simulink model "UPFC"  (R2021a)
settings: Solver=ode45  StartTime=0.0  StopTime=1  RelTol=1e-3  EnableMultiTasking=on
undefined symbols (not defined in the file): D1, Delta
libraries: spsThreePhaseVIMeasurementLib x9, spsMosfetLib x6, spsThyristorLib x6, spsVoltageMeasurementLib x3, spsThreePhaseBreakerLib x2, spsThreePhaseTransformerInductanceMatrixTypeTwoWindingsLib x2, spsCurrentMeasurementLib x1, spsSeriesRLCBranchLib x1, spsDistributedParametersLineLib x1, spsThreePhaseSourceLib x1, spspowerguiLib x1
settings Model: Creator=Indhu  LastModifiedBy=Rahul
settings SolverCC: AlgebraicLoopSolver=TrustRegion
settings DataIOCC: LimitDataPoints=on  SaveFormat=Array  ReturnWorkspaceOutputs=off
settings OptimizationCC: LifeSpan=inf
settings DebuggingCC: SolverPrmCheckMsg=warning  SFUnexpectedBacktrackingDiag=warning  SFNoUnconditionalDefaultTransitionDiag=warning  SFExecutionAtInitializationDiag=none  SFMachineParentedDataDiag=warning  ArithmeticOperatorsInVariantConditions=warning
settings HardwareCC: ProdBitPerPointer=32  ProdBitPerSizeT=32  ProdBitPerPtrDiffT=32  ProdLargestAtomicFloat=None  ProdIntDivRoundTo=Undefined  ProdEndianess=Unspecified  ProdWordSize=32  ProdHWDeviceType=32-bit Generic
settings ModelReferenceCC: PropagateSignalLabelsOutOfModel=off
settings SFSimCC: SimUseLocalCustomCode=off  CustomCodeUndefinedFunction=UseInterfaceOnly
settings RTWCC: RTWUseLocalCustomCode=off
settings CodeAppCC: StateflowObjectComments=on
settings GRTTargetCC: TargetLangStandard=C89/C90 (ANSI)
settings ConfigComp: CovMetricSettings=dw  CovSaveCumulativeToWorkspaceVar=on  CovSaveSingleToWorkspaceVar=on  CovExternalEMLEnable=off  CovSFcnEnable=off
settings SimscapeCC: SimscapeNormalizeSystem=off

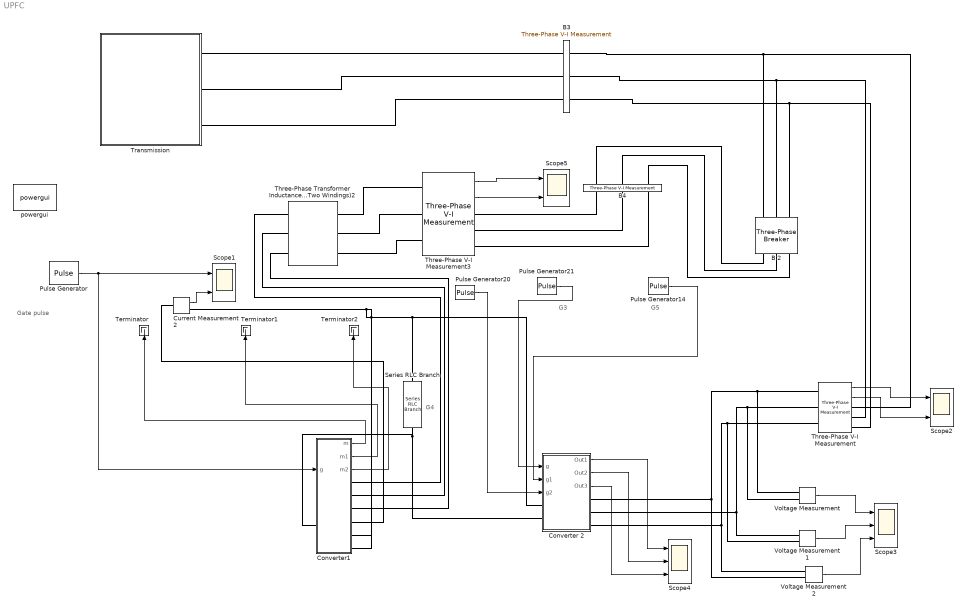
== system UPFC ==
  note: G4
  note: G5
  note: G3
  note: Gate pulse
  B 2 : spsThreePhaseBreakerLib/Three-Phase Breaker  InitialState=closed  SwitchA=off  SwitchB=off  SwitchC=off  SwitchTimes="[1/50  20/50]"  External=off  BreakerResistance=0.001  SnubberResistance=1e6  SnubberCapacitance=inf  Measurements=None
  B3 : spsThreePhaseVIMeasurementLib/Three-Phase V-I Measurement  VoltageMeasurement=phase-to-ground  SetLabelV=on  LabelV=Vabc_B3  Vpu=off  VpuLL=off  CurrentMeasurement=no  SetLabelI=off  LabelI=A1  Ipu=off  Pbase=100e6  Vbase=440  OutputType=Magnitude  PhasorSimulation=off  PSBequivalent=0
  B4 : spsThreePhaseVIMeasurementLib/Three-Phase V-I Measurement  VoltageMeasurement=phase-to-phase  SetLabelV=on  LabelV=Vabc_B4  Vpu=off  VpuLL=off  CurrentMeasurement=yes  SetLabelI=on  LabelI=Iabc_B4  Ipu=off  Pbase=100e6  Vbase=440  OutputType=Magnitude  PhasorSimulation=off  PSBequivalent=0
  Converter 2 : Subsystem
  Converter1 : Subsystem
  Current Measurement2 : spsCurrentMeasurementLib/Current Measurement  PhasorSimulation=off  OutputType=Complex  PSBequivalent=0
  Pulse Generator : DiscretePulseGenerator  PulseType=Time based  Amplitude=10  Period=0.02/3  PulseWidth=20  PhaseDelay=0.0025
  Pulse Generator14 : DiscretePulseGenerator  PulseType=Time based  Period=0.02  PulseWidth=50  PhaseDelay=0.04/3
  Pulse Generator20 : DiscretePulseGenerator  PulseType=Time based  Period=0.02  PulseWidth=50
  Pulse Generator21 : DiscretePulseGenerator  PulseType=Time based  Period=0.02  PulseWidth=50  PhaseDelay=0.02/3
  Scope1 : Scope  NumInputPorts=2
  Scope2 : Scope  NumInputPorts=2
  Scope3 : Scope  NumInputPorts=3
  Scope4 : Scope  NumInputPorts=3
  Scope5 : Scope  NumInputPorts=2
  Series RLC Branch : spsSeriesRLCBranchLib/Series RLC Branch  LConnTagsString=__new0  RConnTagsString=__new0  BranchType=C  Resistance=1  Inductance=1e-3  SetiL0=off  InitialCurrent=0  Capacitance=10  Setx0=off  InitialVoltage=0  Measurements=None
  Terminator : Terminator
  Terminator1 : Terminator
  Terminator2 : Terminator
  Three-Phase V-I Measurement : spsThreePhaseVIMeasurementLib/Three-Phase V-I Measurement  VoltageMeasurement=phase-to-ground  SetLabelV=off  LabelV=Vabc  Vpu=off  VpuLL=off  CurrentMeasurement=yes  SetLabelI=off  LabelI=Iabc  Ipu=off  Pbase=100e6  Vbase=500e3  OutputType=Complex  PhasorSimulation=off  PSBequivalent=0
  Three-Phase V-I Measurement3 : spsThreePhaseVIMeasurementLib/Three-Phase V-I Measurement  VoltageMeasurement=phase-to-phase  SetLabelV=off  LabelV=Vabc  Vpu=off  VpuLL=off  CurrentMeasurement=yes  SetLabelI=off  LabelI=Iabc  Ipu=off  Pbase=100e6  Vbase=500e3  OutputType=Complex  PhasorSimulation=off  PSBequivalent=0
  Three-Phase Transformer Inductance Matrix Type (Two Windings)2 : spsThreePhaseTransformerInductanceMatrixTypeTwoWindingsLib/Three-Phase Transformer Inductance Matrix Type (Two Windings)  CoreType=Three-limb or five-limb core  Winding1Connection=Delta (D1)  Winding2Connection=Yg  AutoTransformer=off  Measurements=None  NominalPower=[100e3 50]  VLLnom=[254.03 254.03]  WindingResistances=[0.01 0.01]  NoLoadIexcPos=2  NoLoadPlossPos=1000  ShortCircuitReactancePos=0.06  ShortCircuitReactancePosAuto=0.06  NoLoadIexcZero=100  NoLoadPlossZero=1500  ShortCircuitReactanceZero=0.03  ShortCircuitReactanceZeroAuto=0.03
      settings: SourceProductBaseCode=PS
  "Transmission " : Subsystem
  Voltage Measurement : spsVoltageMeasurementLib/Voltage Measurement  PhasorSimulation=off  OutputType=Complex  PSBequivalent=0
  Voltage Measurement1 : spsVoltageMeasurementLib/Voltage Measurement  PhasorSimulation=off  OutputType=Complex  PSBequivalent=0
  Voltage Measurement2 : spsVoltageMeasurementLib/Voltage Measurement  PhasorSimulation=off  OutputType=Complex  PSBequivalent=0
  powergui : spspowerguiLib/powergui  Priority=1  SimulationMode=Discrete  SampleTime=50e-6  frequency=60  Iterations=50  frequencyindice=50  Pbase=100e6  ErrMax=1e-4  UnitsV=kV  UnitsW=MW  buscounter=0  FunctionMessages=off  echomessages=off  EnableUseOfTLC=off  CurrentSourceSwitches=off  DisableSnubberDevices=off  DisableRonSwitches=off  DisableVfSwitches=off  DisplayEquations=off  AutomaticDiscreteSolvers=off  SolverType=Tustin  Interpol=off  ExternalGateDelay=off  methode=off  Ts=0  x0status=blocks  SPID=off  SwTol=0  HookPort=off  NonlinearTolerance=1e-4  nMaxIteration=100  ContinueOnMaxIteration=off  RestoreLinks=warning  ResistiveCurrentMeasurement=off  Frange=[0:2:500]  Ylog=off  Xlog=on  ShowGrid=off  save=off  variable=ZData  structure=0  ZoomFFT=off  StartTime=0.0  cycles=1  DisplayStyle=1  fundamental=60  FreqAxis=off  MaxFrequency=1000  frequencyindicesteady=1  RmsSteady=1  display=off
  wires:
  Pulse Generator/1 -> Converter1/1(g), Scope1/1
  Current Measurement2/1 -> Scope1/2
  Three-Phase V-I Measurement/2 -> Scope2/2
  Three-Phase V-I Measurement/1 -> Scope2/1
  Voltage Measurement/1 -> Scope3/1
  Voltage Measurement1/1 -> Scope3/2
  Voltage Measurement2/1 -> Scope3/3
  Three-Phase V-I Measurement3/1 -> Scope5/1
  Three-Phase V-I Measurement3/2 -> Scope5/2
  Converter1/1(m) -> Terminator/1
  Converter1/2(m1) -> Terminator1/1
  Converter1/3(m2) -> Terminator2/1
  Pulse Generator21/1 -> Converter 2/1(g)
  Pulse Generator14/1 -> Converter 2/2(g1)
  Pulse Generator20/1 -> Converter 2/3(g2)
  Converter 2/1(Out1) -> Scope4/1
  Converter 2/2(Out2) -> Scope4/2
  Converter 2/3(Out3) -> Scope4/3
  connections:
  Current Measurement2/RConn1 -- Converter1/RConn5 -- Converter1/RConn6 -- Converter 2/LConn1 -- Series RLC Branch/LConn1
  Series RLC Branch/RConn1 -- Converter 2/LConn2 -- Converter1/LConn1
  Voltage Measurement1/LConn1 -- Voltage Measurement/LConn2 -- Three-Phase V-I Measurement/LConn2 -- Converter 2/RConn2
  B3/LConn3 -- Three-Phase V-I Measurement/RConn3 -- B 2/LConn3
  B3/LConn1 -- Three-Phase V-I Measurement/RConn1 -- B 2/LConn1
  B3/LConn2 -- Three-Phase V-I Measurement/RConn2 -- B 2/LConn2
  Three-Phase V-I Measurement3/RConn3 -- B4/RConn3
  B4/LConn1 -- B 2/RConn1
  B4/LConn3 -- B 2/RConn3
  Three-Phase V-I Measurement3/RConn1 -- B4/RConn1
  Three-Phase V-I Measurement3/RConn2 -- B4/RConn2
  B4/LConn2 -- B 2/RConn2
  Three-Phase V-I Measurement3/LConn1 -- Three-Phase Transformer Inductance Matrix Type (Two Windings)2/RConn1
  Three-Phase V-I Measurement3/LConn2 -- Three-Phase Transformer Inductance Matrix Type (Two Windings)2/RConn2
  Three-Phase V-I Measurement3/LConn3 -- Three-Phase Transformer Inductance Matrix Type (Two Windings)2/RConn3
  Three-Phase Transformer Inductance Matrix Type (Two Windings)2/LConn1 -- Converter1/RConn1
  Three-Phase Transformer Inductance Matrix Type (Two Windings)2/LConn2 -- Converter1/RConn2
  Three-Phase Transformer Inductance Matrix Type (Two Windings)2/LConn3 -- Converter1/RConn3
  Current Measurement2/LConn1 -- Converter1/RConn4
  Voltage Measurement2/LConn2 -- Voltage Measurement/LConn1 -- Three-Phase V-I Measurement/LConn1 -- Converter 2/RConn1
  Voltage Measurement1/LConn2 -- Voltage Measurement2/LConn1 -- Converter 2/RConn3 -- Three-Phase V-I Measurement/LConn3
  "Transmission "/RConn1 -- B3/RConn1
  "Transmission "/RConn2 -- B3/RConn2
  "Transmission "/RConn3 -- B3/RConn3

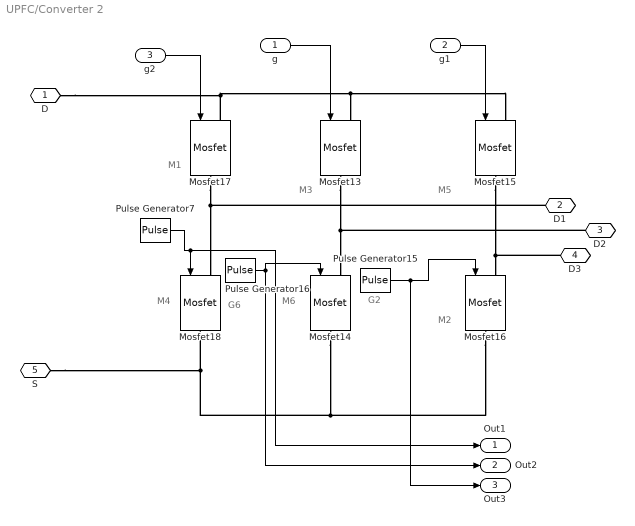
== system UPFC/Converter 2 ==
  note: M1
  note: M2
  note: M4
  note: M6
  note: M3
  note: M5
  note: G6
  note: G2
  g : Inport
  g1 : Inport  Port=2
  g2 : Inport  Port=3
  Mosfet{13..18} (6 alike) : spsMosfetLib/Mosfet  Ron=0.001  Lon=1e-6  Rd=.001  Vfd=0  IC=0  Rs=1e5  Cs=inf  Measurements=off
  Pulse Generator15 : DiscretePulseGenerator  PulseType=Time based  Period=0.02  PulseWidth=50  PhaseDelay=0.01/3
  Pulse Generator16 : DiscretePulseGenerator  PulseType=Time based  Period=0.02  PulseWidth=50  PhaseDelay=0.05/3
  Pulse Generator7 : DiscretePulseGenerator  PulseType=Time based  Period=0.02  PulseWidth=50  PhaseDelay=0.01
  D : PMIOPort  Side=Left
  D1 : PMIOPort  Port=2  Side=Right
  D2 : PMIOPort  Port=3  Side=Right
  D3 : PMIOPort  Port=4  Side=Right
  S : PMIOPort  Port=5  Side=Left
  Out1 : Outport
  Out2 : Outport  Port=2
  Out3 : Outport  Port=3
  wires:
  Pulse Generator7/1 -> Out1/1, Mosfet18/1
  Pulse Generator15/1 -> Out3/1, Mosfet16/1
  g1/1 -> Mosfet15/1
  Pulse Generator16/1 -> Out2/1, Mosfet14/1
  g/1 -> Mosfet13/1
  g2/1 -> Mosfet17/1
  connections:
  Mosfet17/LConn1 -- Mosfet15/LConn1 -- Mosfet13/LConn1 -- D/RConn1
  Mosfet16/RConn1 -- S/RConn1 -- Mosfet18/RConn1 -- Mosfet14/RConn1
  Mosfet17/RConn1 -- D1/RConn1 -- Mosfet18/LConn1
  Mosfet13/RConn1 -- D2/RConn1 -- Mosfet14/LConn1
  Mosfet15/RConn1 -- D3/RConn1 -- Mosfet16/LConn1

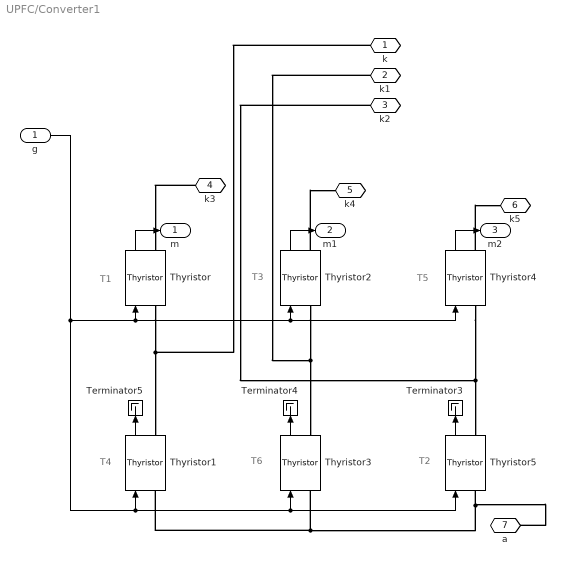
== system UPFC/Converter1 ==
  note: T1
  note: T4
  note: T3
  note: T5
  note: T6
  note: T2
  g : Inport
  Terminator3 : Terminator
  Terminator4 : Terminator
  Terminator5 : Terminator
  Thyristor{,1..5} (6 alike) : spsThyristorLib/Thyristor  Ron=0.001  Lon=0  Vf=0.8  IC=0  Rs=500  Cs=250e-9  Measurements=on
  k : PMIOPort  Side=Right
  k1 : PMIOPort  Port=2  Side=Right
  k2 : PMIOPort  Port=3  Side=Right
  k3 : PMIOPort  Port=4  Side=Right
  k4 : PMIOPort  Port=5  Side=Right
  k5 : PMIOPort  Port=6  Side=Right
  a : PMIOPort  Port=7  Side=Left
  m : Outport
  m1 : Outport  Port=2
  m2 : Outport  Port=3
  wires:
  Thyristor3/1 -> Terminator4/1
  Thyristor5/1 -> Terminator3/1
  g/1 -> Thyristor1/1, Thyristor5/1, Thyristor3/1, Thyristor/1, Thyristor2/1, Thyristor4/1
  Thyristor1/1 -> Terminator5/1
  Thyristor4/1 -> m2/1
  Thyristor/1 -> m/1
  Thyristor2/1 -> m1/1
  connections:
  Thyristor4/LConn1 -- k2/RConn1 -- Thyristor5/RConn1
  Thyristor5/LConn1 -- Thyristor1/LConn1 -- Thyristor3/LConn1 -- a/RConn1
  Thyristor2/LConn1 -- k1/RConn1 -- Thyristor3/RConn1
  Thyristor/LConn1 -- k/RConn1 -- Thyristor1/RConn1
  k3/RConn1 -- Thyristor/RConn1
  Thyristor2/RConn1 -- k4/RConn1
  Thyristor4/RConn1 -- k5/RConn1

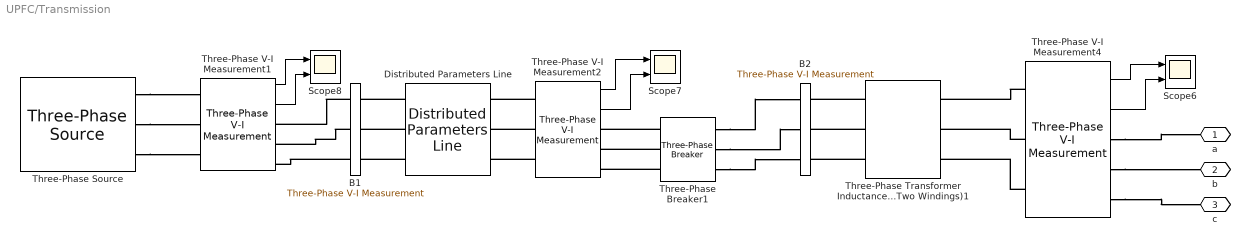
== system UPFC/Transmission  ==
  B1 : spsThreePhaseVIMeasurementLib/Three-Phase V-I Measurement  VoltageMeasurement=phase-to-ground  SetLabelV=on  LabelV=Vabc_B1  Vpu=off  VpuLL=off  CurrentMeasurement=no  SetLabelI=off  LabelI=A1  Ipu=off  Pbase=100e6  Vbase=25e3  OutputType=Magnitude  PhasorSimulation=off  PSBequivalent=0
  B2 : spsThreePhaseVIMeasurementLib/Three-Phase V-I Measurement  VoltageMeasurement=phase-to-ground  SetLabelV=on  LabelV=Vabc_B2  Vpu=off  VpuLL=off  CurrentMeasurement=no  SetLabelI=off  LabelI=A1  Ipu=off  Pbase=100e6  Vbase=440  OutputType=Magnitude  PhasorSimulation=off  PSBequivalent=0
  Distributed Parameters Line : spsDistributedParametersLineLib/Distributed Parameters Line  Phases=3  Length=100  Frequency=50  Resistance=[0.01273 0.3864]  Inductance="[0.9337e-3  4.1264e-3]"  Capacitance=[12.74e-9 7.751e-9]  x1=[-0.0006 5.86839207173151e-09 21084.9928612952 -61013.4621730044;-0.00055 5.88763685316343e-09 22040.7494686959 -60674.7464202009;-0.0005 5.90542894830042e-09 22991.0678509681 -60321.0600816139;-0.00045 5.92176396720926e-09 23935.7135312707 -59952.4904240552;-0.0004 5.93663787946844e-09 24874.4534324173 -59569.1283865727;-0.00035 5.95004701516269e-09 25807.0559343838 -59171.0685580128;-0.0003 5.9619880657884e-09 26733.2909314579 -58758.4091536819;-0.00025 5.97245808507003e-09 27652.9298890134 -58331.2519911133;-0.0002 5.98145448968697e-09 28565.7458998984 -57889.7024649452;-0.00015 5.98897505991101e-09 29471.5137404211 -57433.8695209161;-0.0001 5.99501794015397e-09 30370.0099259201 -56963.8656289841;-5e-05 5.99958163942558e-09 31261.012765906 -56479.8067555767]  x2=[-0.0006 2.43838460320936e-08 21192.2989946468 -61377.500589569;-0.00055 2.45095717766997e-08 22153.7604308789 -61037.0544347634;-0.0005 2.46292501512145e-08 23109.7557582185 -60681.548300093;-0.00045 2.47428516267898e-08 24060.0490991234 -60311.069901377;-0.0004 2.48503481739615e-08 25004.4059829314 -59925.7106486168;-0.00035 2.4951713269565e-08 25942.5934037121 -59525.5656234417;-0.0003 2.50469219032797e-08 26874.3798777577 -59110.7335556492;-0.00025 2.51359505838e-08 27799.5355006985 -58681.3167988447;-0.0002 2.52187773446309e-08 28717.8320042279 -58237.4213051875;-0.00015 2.52953817495088e-08 29629.0428124244 -57779.1565992484;-0.0001 2.53657448974429e-08 30532.9430976558 -57306.6357509866;-5e-05 2.54298494273793e-08 31429.309836052 -56819.9753478508]  x3=[-0.0006 -2.39104500674847e-12 53.1931047383557 -232.981131649146;-0.00055 -1.12649559613069e-13 56.8460509995095 -232.116868370186;-0.0005 2.16577368211556e-12 60.484971348185 -231.195333727194;-0.00045 4.44366255159529e-12 64.1089679352363 -230.216755095056;-0.0004 6.72045501383237e-12 67.7171465937327 -229.181373923405;-0.00035 8.99558930435511e-12 71.3086170595806 -228.089445677053;-0.0003 1.12685040678209e-11 74.8824931911827 -226.941239772955;-0.00025 1.35386384965222e-11 78.4378931880807 -225.737039513739;-0.0002 1.58054324687575e-11 81.9739398085259 -224.477142017798;-0.00015 1.80683266870328e-11 85.4897605859257 -223.161858145988;-0.0001 2.03267628160604e-11 88.9844880441118 -221.791512424923;-5e-05 2.25801836205189e-11 92.4572599113764 -220.366442966905]  x4=[-0.0006 4.11118395045662e-11 77.9640644175601 -225.970631131285;-0.00055 3.90812302073656e-11 81.5038385907474 -224.71814739658;-0.0005 3.70409782013962e-11 85.0235029113307 -223.410217821535;-0.00045 3.49915868883118e-11 88.5221889548044 -222.047165118202;-0.0004 3.29335619247529e-11 91.9990334727396 -220.629325599439;-0.00035 3.08674110975847e-11 95.4531786057765 -219.157049095931;-0.0003 2.8793644198607e-11 98.8837720952889 -217.630698869876;-0.00025 2.6712772898772e-11 102.289967493667 -216.050651525354;-0.0002 2.46253106219359e-11 105.670924373163 -214.417296915402;-0.00015 2.25317724181803e-11 109.025808533258 -212.731038045832;-0.0001 2.04326748367307e-11 112.353792206485 -210.992290975787;-5e-05 1.83285357985058e-11 115.654054262672 -209.201484715089]  x5=0.000565541566995743  V1=ones(3,3)  V2=ones(3,3)  I1=ones(3,3)  I2=ones(3,3)  nHarmo=1  Measurements=None  Decoupling=off  VsMag0=0  VrMag0=0  VsAngle0=0  VrAngle0=0  IsMag0=0  IrMag0=0  IsAngle0=0  IrAngle0=0
      settings: SourceProductBaseCode=PS
  Scope6 : Scope  NumInputPorts=2
  Scope7 : Scope  NumInputPorts=2
  Scope8 : Scope  NumInputPorts=2
  Three-Phase V-I Measurement1 : spsThreePhaseVIMeasurementLib/Three-Phase V-I Measurement  VoltageMeasurement=phase-to-ground  SetLabelV=off  LabelV=Vabc  Vpu=off  VpuLL=off  CurrentMeasurement=yes  SetLabelI=off  LabelI=Iabc  Ipu=off  Pbase=100e6  Vbase=500e3  OutputType=Complex  PhasorSimulation=off  PSBequivalent=0
  Three-Phase V-I Measurement2 : spsThreePhaseVIMeasurementLib/Three-Phase V-I Measurement  VoltageMeasurement=phase-to-ground  SetLabelV=off  LabelV=Vabc  Vpu=off  VpuLL=off  CurrentMeasurement=yes  SetLabelI=off  LabelI=Iabc  Ipu=off  Pbase=100e6  Vbase=500e3  OutputType=Complex  PhasorSimulation=off  PSBequivalent=0
  Three-Phase V-I Measurement4 : spsThreePhaseVIMeasurementLib/Three-Phase V-I Measurement  VoltageMeasurement=phase-to-ground  SetLabelV=off  LabelV=Vabc  Vpu=off  VpuLL=off  CurrentMeasurement=yes  SetLabelI=off  LabelI=Iabc  Ipu=off  Pbase=100e6  Vbase=500e3  OutputType=Complex  PhasorSimulation=off  PSBequivalent=0
  Three-Phase Breaker1 : spsThreePhaseBreakerLib/Three-Phase Breaker  InitialState=closed  SwitchA=off  SwitchB=off  SwitchC=off  SwitchTimes="[1/50  20/50]"  External=off  BreakerResistance=0.001  SnubberResistance=1e6  SnubberCapacitance=inf  Measurements=None
  Three-Phase Source : spsThreePhaseSourceLib/Three-Phase Source  InternalConnection=Yg  VoltagePhases=off  Voltage=63510.4  PhaseAngle=0  Voltage_phases=[25e3 25e3 25e3]/sqrt(3)  PhaseAngles_phases=[0 -120 +120]  Frequency=50  NonIdealSource=on  SpecifyImpedance=on  Resistance=0.8929  Inductance=16.58e-3  ShortCircuitLevel=100e6  BaseVoltage=63510.4  XRratio=7  BusType=swing  Pref=0  Qref=0  Prefabc=[10e3, 10e3, 10e3]  Qrefabc=[0, 0, 0]  Qmin=-inf  Qmax=inf
  Three-Phase Transformer Inductance Matrix Type (Two Windings)1 : spsThreePhaseTransformerInductanceMatrixTypeTwoWindingsLib/Three-Phase Transformer Inductance Matrix Type (Two Windings)  CoreType=Three-limb or five-limb core  Winding1Connection=Yg  Winding2Connection=Yg  AutoTransformer=off  Measurements=None  NominalPower=[100e3 50]  VLLnom=[63510.4 254.03]  WindingResistances=[0.01 0.01]  NoLoadIexcPos=2  NoLoadPlossPos=1000  ShortCircuitReactancePos=0.06  ShortCircuitReactancePosAuto=0.06  NoLoadIexcZero=100  NoLoadPlossZero=1500  ShortCircuitReactanceZero=0.03  ShortCircuitReactanceZeroAuto=0.03
      settings: SourceProductBaseCode=PS
  a : PMIOPort  Side=Right
  b : PMIOPort  Port=2  Side=Right
  c : PMIOPort  Port=3  Side=Right
  wires:
  Three-Phase V-I Measurement2/1 -> Scope7/1
  Three-Phase V-I Measurement2/2 -> Scope7/2
  Three-Phase V-I Measurement1/2 -> Scope8/2
  Three-Phase V-I Measurement4/1 -> Scope6/1
  Three-Phase V-I Measurement1/1 -> Scope8/1
  Three-Phase V-I Measurement4/2 -> Scope6/2
  connections:
  Three-Phase Breaker1/RConn2 -- Three-Phase V-I Measurement2/RConn2
  Three-Phase Transformer Inductance Matrix Type (Two Windings)1/LConn2 -- B2/LConn2
  B1/RConn2 -- Three-Phase V-I Measurement1/RConn2
  Three-Phase Source/RConn2 -- Three-Phase V-I Measurement1/LConn2
  Three-Phase Breaker1/LConn2 -- B2/RConn2
  Three-Phase Transformer Inductance Matrix Type (Two Windings)1/LConn3 -- B2/LConn3
  Three-Phase Breaker1/RConn1 -- Three-Phase V-I Measurement2/RConn1
  Three-Phase V-I Measurement4/LConn3 -- Three-Phase Transformer Inductance Matrix Type (Two Windings)1/RConn3
  Three-Phase V-I Measurement4/RConn3 -- c/RConn1
  Three-Phase Breaker1/LConn3 -- B2/RConn3
  Three-Phase Breaker1/LConn1 -- B2/RConn1
  Three-Phase Breaker1/RConn3 -- Three-Phase V-I Measurement2/RConn3
  B1/RConn1 -- Three-Phase V-I Measurement1/RConn1
  Distributed Parameters Line/LConn3 -- B1/LConn3
  Three-Phase Transformer Inductance Matrix Type (Two Windings)1/LConn1 -- B2/LConn1
  Three-Phase V-I Measurement4/RConn1 -- a/RConn1
  Three-Phase V-I Measurement4/LConn1 -- Three-Phase Transformer Inductance Matrix Type (Two Windings)1/RConn1
  Three-Phase V-I Measurement2/LConn2 -- Distributed Parameters Line/RConn2
  Three-Phase V-I Measurement2/LConn3 -- Distributed Parameters Line/RConn3
  Distributed Parameters Line/LConn1 -- B1/LConn1
  Three-Phase V-I Measurement2/LConn1 -- Distributed Parameters Line/RConn1
  Three-Phase Source/RConn1 -- Three-Phase V-I Measurement1/LConn1
  Three-Phase Source/RConn3 -- Three-Phase V-I Measurement1/LConn3
  B1/RConn3 -- Three-Phase V-I Measurement1/RConn3
  Three-Phase V-I Measurement4/RConn2 -- b/RConn1
  Three-Phase V-I Measurement4/LConn2 -- Three-Phase Transformer Inductance Matrix Type (Two Windings)1/RConn2
  Distributed Parameters Line/LConn2 -- B1/LConn2
